simulink model "Prac_2_Q4"  (R2020a)
settings: Solver=VariableStepAuto  StartTime=0.0  StopTime=10.0  RelTol=1e-3
settings Model: Creator=kaibr  LastModifiedBy=kaibr

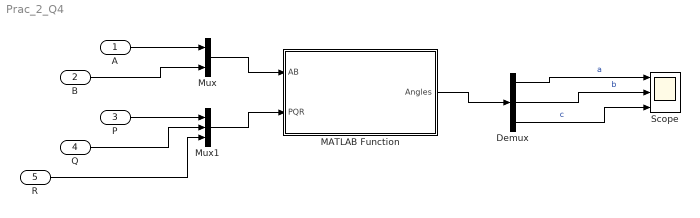
== system Prac_2_Q4 ==
  A : Inport
  B : Inport  Port=2
  P : Inport  Port=3
  Q : Inport  Port=4
  R : Inport  Port=5
  Demux : Demux  Outputs=3
  MATLAB Function : MATLAB Function  TreatAsAtomicUnit=on
  Mux : Mux  Inputs=2
  Mux1 : Mux  Inputs=3
  Scope : Scope  NumInputPorts=3
  wires:
  Mux/1 -> MATLAB Function/1(AB)
  Mux1/1 -> MATLAB Function/2(PQR)
  A/1 -> Mux/1
  B/1 -> Mux/2
  P/1 -> Mux1/1
  Q/1 -> Mux1/2
  R/1 -> Mux1/3
  MATLAB Function/1(Angles) -> Demux/1
  Demux/1 -> Scope/1  "a"
  Demux/2 -> Scope/2  "b"
  Demux/3 -> Scope/3  "c"

== matlab function Prac_2_Q4/MATLAB Function ==
  data: AB input; PQR input; Angles output
function Angles  = eulerMatrix(AB, PQR)
a = AB(1);
b = AB(2);

stateSpace = [
    1 sin(a)*cos(b) cos(a)*tan(b);
    0 cos(a) -sin(a);
    0 sin(a)*sec(b) cos(a)*sec(b)
    ];

Angles = PQR*stateSpace;

end

stateSpace = [
    1 sin(a)*cos(b) cos(a)*tan(b);
    0 cos(a) -sin(a);
    0 sin(a)*sec(b) cos(a)*sec(b)
    ];
